simulink model "step7_steady_state"  (R2025a)
settings: Solver=ode45  StartTime=0.0  StopTime=5  MaxStep=0.01  RelTol=1e-3
undefined symbols (not defined in the file or in its folder): A, B, F, K
settings Model: Creator=O M E N  LastModifiedBy=O M E N

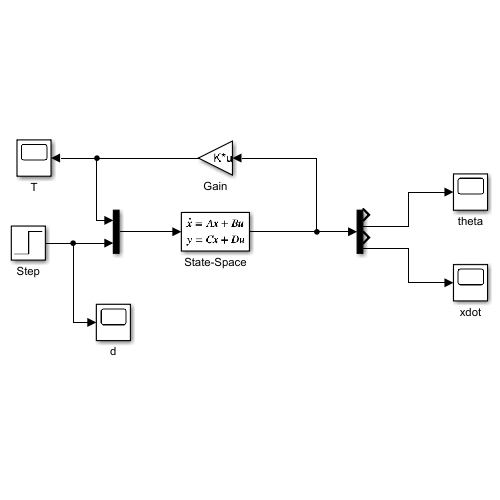
[thumbnail: Simulink's stored preview of the top-level diagram]
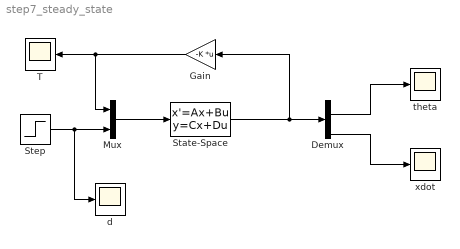
== system step7_steady_state ==
  Demux : Demux
  Gain : Gain  Gain=-K  Multiplication=Matrix(K*u)
  Mux : Mux  Inputs=2
  State-Space : StateSpace  A=A  B=[B F]  C=eye(4)  D=zeros(4,2)  InitialCondition=[0; 0; 0; 0]
  Step : Step  After=0.001  SampleTime=0
  T : Scope
      settings: Title=Control torque T(t)  ActiveDisplayYMinimum=-30.761290876154277  ActiveDisplayYMaximum=38.538057129133136  YLabel="T  (N·m)"  DataLoggingVariableName=ScopeData2
  d : Scope
      settings: Title=Disturbance d(t)  ActiveDisplayYMinimum=-0.0012499999999999998  ActiveDisplayYMaximum=0.01125  YLabel="d  (m)"  DataLoggingVariableName=ScopeData3
  theta : Scope
      settings: Title=Tilt angle θ(t)  ActiveDisplayYMinimum=-0.0020734413320211056  ActiveDisplayYMaximum=0.018218244870607334  YLabel="θ  (rad)"
  xdot : Scope
      settings: Title=Vehicle speed ẋ(t)  ActiveDisplayYMinimum=-0.12679773976405423  ActiveDisplayYMaximum=0.31923072377038231  YLabel="ẋ  (m/s)"
  wires:
  Mux/1 -> State-Space/1
  State-Space/1 -> Gain/1, Demux/1
  Demux/2 -> theta/1
  Demux/4 -> xdot/1
  Gain/1 -> T/1, Mux/1
  Step/1 -> d/1, Mux/2
